simulink model "burst_test"  (R2015b)
settings: Solver=VariableStepAuto  StartTime=0.0  StopTime=10.0  RelTol=1e-3
settings Model: Creator=rajiv  LastModifiedBy=rajiv

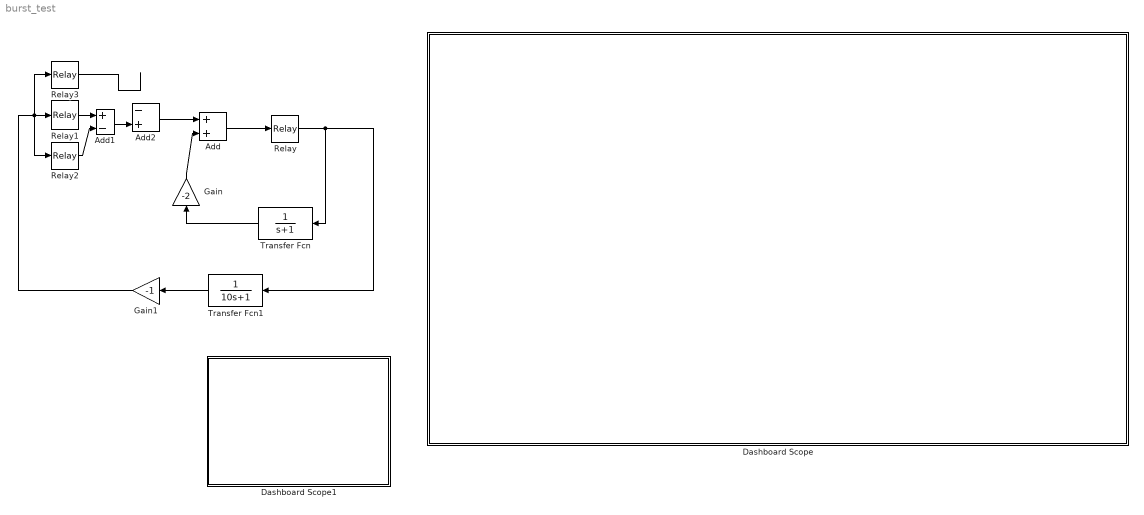
== system burst_test ==
  Add : Sum
  Add1 : Sum  Inputs=+-
  Add2 : Sum  Inputs=-+
  Dashboard Scope : Subsystem  DialogController=hmiCreateDDGDialog  IsWebBlock=on  mask(MWDashboardBlock){webBlockId=91b4fd2c-1a98-4280-95f0-d2fc1d5cc94e, webBlockType=sdiscope, ShowInitialText=on, HMISrcModelName=untitled}
      mask prompts: webBlockId "WebBlock Id"; webBlockType "WebBlock Type"; HMISrcModelName "Source Model"
      mask Help: helpview([docroot '/mapfiles/simulink.map'], 'hmi_scope')
      mask Display:
      | if strcmp(get_param(bdroot(gcb),'BlockDiagramType'), 'library')
      |     image([(matlabroot) '/toolbox/simulink/hmi/icons/DashboardScope.png']);
      | end
  Dashboard Scope1 : Subsystem  DialogController=hmiCreateDDGDialog  IsWebBlock=on  mask(MWDashboardBlock){webBlockId=2a836dc5-d8b5-4fb6-b538-deab662753af, webBlockType=sdiscope, ShowInitialText=on, HMISrcModelName=untitled}
      mask prompts: webBlockId "WebBlock Id"; webBlockType "WebBlock Type"; HMISrcModelName "Source Model"
      mask Help: helpview([docroot '/mapfiles/simulink.map'], 'hmi_scope')
      mask Display:
      | if strcmp(get_param(bdroot(gcb),'BlockDiagramType'), 'library')
      |     image([(matlabroot) '/toolbox/simulink/hmi/icons/DashboardScope.png']);
      | end
  Gain : Gain  Gain=-2
  Gain1 : Gain  Gain=-1
  Relay : Relay  OnSwitchValue=0  OffSwitchValue=-0  OnOutputValue=.1  OffOutputValue=-.1
  Relay1 : Relay  OnSwitchValue=-1  OffSwitchValue=-1  OffOutputValue=-1
  Relay2 : Relay  OnSwitchValue=1  OffSwitchValue=1  OffOutputValue=-1
  Relay3 : Relay  OnSwitchValue=0  OffSwitchValue=0  OnOutputValue=2  OffOutputValue=-2
  Transfer Fcn : TransferFcn  Denominator=[1 1]
  Transfer Fcn1 : TransferFcn  Denominator=[10 1]
  wires:
  Relay/1 -> Transfer Fcn1/1, Transfer Fcn/1
  Transfer Fcn/1 -> Gain/1
  Gain/1 -> Add/2
  Add/1 -> Relay/1
  Relay2/1 -> Add1/2
  Relay1/1 -> Add1/1
  Add1/1 -> Add2/2
  Relay3/1 -> ?
  Transfer Fcn1/1 -> Gain1/1
  Gain1/1 -> Relay2/1, Relay3/1, Relay1/1
  Add2/1 -> Add/1

== system burst_test/Dashboard Scope ==

== system burst_test/Dashboard Scope1 ==
